simulink model "SimpleModel"  (R2020b)
settings: Solver=VariableStepAuto  StartTime=0.0  StopTime=10.0  RelTol=1e-3
undefined symbols (not defined in the file): A, B, C, D
libraries: simulink x1
settings Model: Creator=karshenas  LastModifiedBy=karshenas

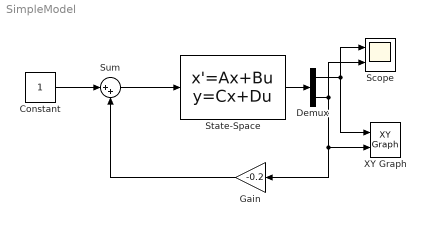
== system SimpleModel ==
  Constant : Constant
  Demux : Demux  Outputs=2
  Gain : Gain  Gain=-0.2
  Scope : Scope  NumInputPorts=2
  State-Space : StateSpace  A=A  B=B  C=C  D=D  InitialCondition=0
  Sum : Sum  Inputs=|++
  XY Graph : simulink/Sinks/XY Graph  xmin=-1  xmax=1  ymin=-1  ymax=1  st=-1
  wires:
  State-Space/1 -> Demux/1
  Demux/1 -> XY Graph/1, Scope/1
  Demux/2 -> Gain/1, XY Graph/2, Scope/2
  Constant/1 -> Sum/1
  Gain/1 -> Sum/2
  Sum/1 -> State-Space/1
